simulink model "ip_1"  (Simulink 5.0)
settings: Solver=ode5  SolverMode=SingleTasking  StartTime=0.0  StopTime=inf  RelTol=1e-3
libraries: pci1711 x3
settings Model: LastModifiedBy=AD  ExtModeMexFile=rtwinext  SimulationMode=external  BooleanDataType=off  RTWSystemTargetFile=rtwin.tlc  RTWTemplateMakefile=rtwintmf  RTWOptions="-aCCOptimize=1 -aEnforceIntegerDowncast=1 -aExtMode=0 -aFoldNonRolledExpr=1 -aForceParamTrailComments=0 -aGenerateComments=1 -aGenerateReport=0 -aIncDataTypeInIds=0 -aIncHierarchyInIds=0 -aInlineInvariantSignals=0 -aInlineParameters=0 -aInlinedPrmAccess=\"Literals\" -aLocalBlockOutputs=1 -aMaxRTWIdLen=31 -aPrefixModelToSubsysFcnNames=1 -aRTWVerbose=1 -aRebuildAll=0 -aRollThreshold=5 -aShowEliminatedStatements=0"

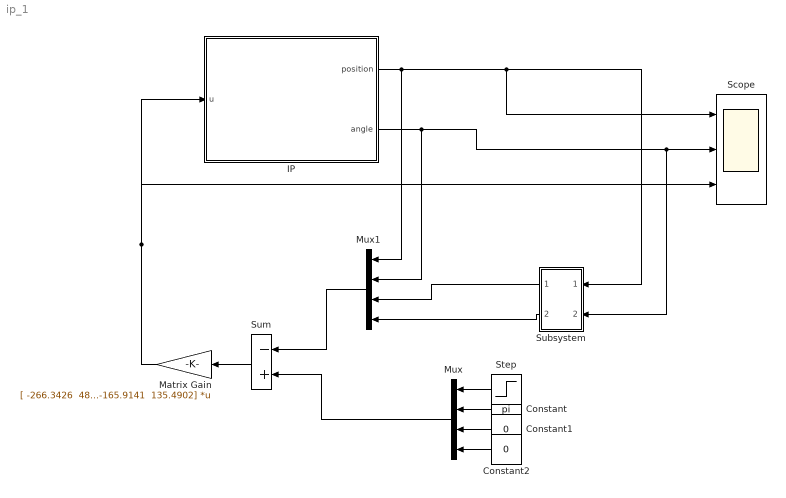
== system ip_1 ==
  Constant : Constant  Orientation=left  Value=pi
  Constant1 : Constant  Orientation=left  Value=0
  Constant2 : Constant  Orientation=left  Value=0
  IP : Subsystem
  Matrix Gain : Gain  Orientation=left  Gain="[ -266.3426  481.7491 -165.9141  135.4902]"  Multiplication=Matrix(K*u)  SaturateOnIntegerOverflow=on
  Mux : Mux  Orientation=left
  Mux1 : Mux  Orientation=left
  Scope : Scope  NumInputPorts=3
      settings: TickLabels=on  TimeRange=50  YMin=0.0557197~3.03989~-2.6292  YMax=0.0615849~3.35987~-2.3788  Decimation=10  SampleInput=on  SampleTime=0.01
  Step : Step  Orientation=left  Time=10  After=0  SampleTime=0
  Subsystem : Subsystem  Orientation=left
  Sum : Sum  Orientation=left  Inputs=-+  SaturateOnIntegerOverflow=on
  wires:
  IP/1(position) -> Subsystem/1(In1), Scope/1, Mux1/1
  IP/2(angle) -> Mux1/2, Subsystem/2(In2), Scope/2
  Step/1 -> Mux/1
  Constant/1 -> Mux/2
  Constant1/1 -> Mux/3
  Constant2/1 -> Mux/4
  Mux1/1 -> Sum/1
  Mux/1 -> Sum/2
  Sum/1 -> Matrix Gain/1
  Matrix Gain/1 -> Scope/3, IP/1(u)
  Subsystem/2(Out2) -> Mux1/4
  Subsystem/1(Out1) -> Mux1/3

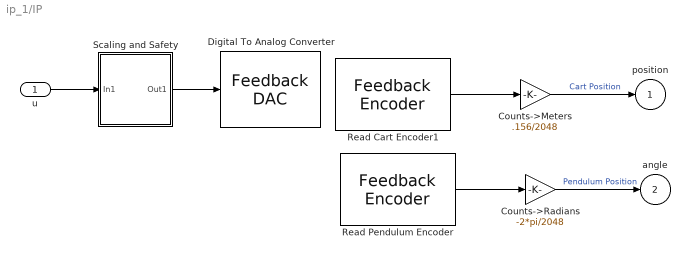
== system ip_1/IP ==
  u : Inport
  Counts->Meters : Gain  Gain=.156/2048  SaturateOnIntegerOverflow=on
  Counts->Radians : Gain  Gain=-2*pi/2048  SaturateOnIntegerOverflow=on
  Digital To Analog Converter : pci1711/Advantech  PCI1711 I//O Board Lib/Feedback DAC  channel=0  range=0  tsamp=0.001  hwAccess=on
  Read Cart Encoder1 : pci1711/Advantech  PCI1711 I//O Board Lib/Feedback Encoder   channel=0  offset=0  tsamp=0.001  hwAccess=on
  Read Pendulum Encoder : pci1711/Advantech  PCI1711 I//O Board Lib/Feedback Encoder   channel=1  offset=-1024  tsamp=0.001  hwAccess=on
  Scaling and Safety : Subsystem
  position : Outport
  angle : Outport  Port=2
  wires:
  Scaling and Safety/1(Out1) -> Digital To Analog Converter/1
  u/1 -> Scaling and Safety/1(In1)
  Read Cart Encoder1/1 -> Counts->Meters/1
  Read Pendulum Encoder/1 -> Counts->Radians/1
  Counts->Radians/1 -> angle/1  "Pendulum Position"
  Counts->Meters/1 -> position/1  "Cart Position"

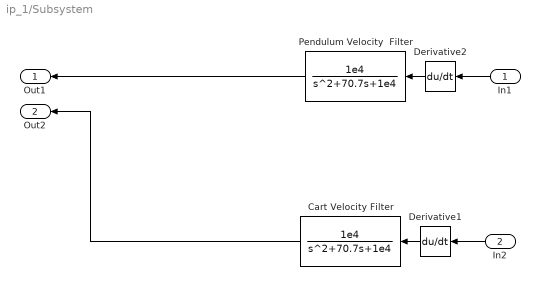
== system ip_1/Subsystem ==
  In1 : Inport  Orientation=left
  In2 : Inport  Orientation=left  Port=2
  Cart Velocity Filter : TransferFcn  Orientation=left  Numerator=[1e4]  Denominator=[1 70.7 1e4]
  Derivative1 : Derivative  Orientation=left
  Derivative2 : Derivative  Orientation=left
  Pendulum Velocity  Filter : TransferFcn  Orientation=left  Numerator=[1e4]  Denominator=[1 70.7 1e4]
  Out1 : Outport  Orientation=left
  Out2 : Outport  Orientation=left  Port=2
  wires:
  Cart Velocity Filter/1 -> Out2/1
  Pendulum Velocity  Filter/1 -> Out1/1
  In2/1 -> Derivative1/1
  In1/1 -> Derivative2/1
  Derivative1/1 -> Cart Velocity Filter/1
  Derivative2/1 -> Pendulum Velocity  Filter/1

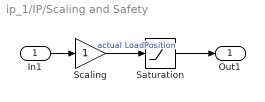
== system ip_1/IP/Scaling and Safety ==
  In1 : Inport
  Saturation : Saturate  UpperLimit=2.5  LowerLimit=-2.5
  Scaling : Gain  SaturateOnIntegerOverflow=on
  Out1 : Outport
  wires:
  Scaling/1 -> Saturation/1  "actual LoadPosition"
  In1/1 -> Scaling/1
  Saturation/1 -> Out1/1
